simulink model "Kunal-Jain_14AE10019_MagLev"  (R2015a)
settings: Solver=ode23  StartTime=0.0  StopTime=10  RelTol=1e-3
libraries: simulink x4
settings Model: Creator=Kunal  LastModifiedBy=Kunal
settings SolverCC: AutoInsertRateTranBlk=on

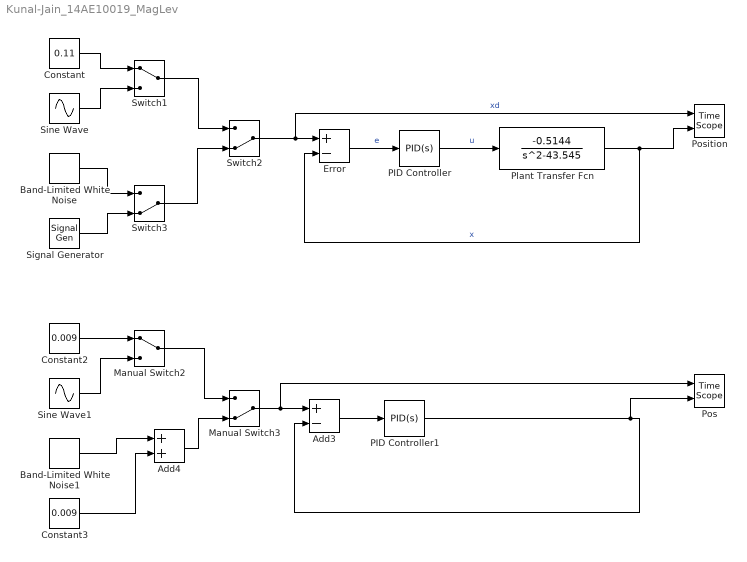
== system Kunal-Jain_14AE10019_MagLev ==
  Add3 : Sum  Inputs=+-
  Add4 : Sum
  Band-Limited White Noise : simulink/Sources/Band-Limited White Noise  Cov=[0.1]  Ts=0.1  seed=[23341]
  Band-Limited White Noise1 : simulink/Sources/Band-Limited White Noise  Cov=[0.1]  Ts=0.1  seed=[23341]
  Constant : Constant  Value=0.11
  Constant2 : Constant  Value=0.009
  Constant3 : Constant  Value=0.009
  Error : Sum  Inputs=+-
  Manual Switch2 : ManualSwitch
  Manual Switch3 : ManualSwitch  CurrentSetting=0
  PID Controller : simulink/Continuous/PID Controller  Controller=PID  TimeDomain=Continuous-time  SampleTime=-1  IntegratorMethod=Forward Euler  FilterMethod=Forward Euler  Form=Parallel  UseFilter=on  ControllerParametersSource=internal  P=-1802.63633168845  I=-5937.61734268954  D=-134.383925464391  N=383.737180014477  InitialConditionSource=internal  InitialConditionForIntegrator=0  InitialConditionForFilter=0  ExternalReset=none  LimitOutput=off  UpperSaturationLimit=inf  LowerSaturationLimit=-inf  LinearizeAsGain=on  AntiWindupMode=none  Kb=1  TrackingMode=off  Kt=1  PParamMin=[]  PParamMax=[]  IParamMin=[]  IParamMax=[]  DParamMin=[]  DParamMax=[]  NParamMin=[]  NParamMax=[]  KbParamMin=[]  KbParamMax=[]  KtParamMin=[]  KtParamMax=[]  POutMin=[]  POutMax=[]  IOutMin=[]  IOutMax=[]  DOutMin=[]  DOutMax=[]  NOutMin=[]  NOutMax=[]  KbOutMin=[]  KbOutMax=[]  KtOutMin=[]  KtOutMax=[]  IntegratorOutMin=[]  IntegratorOutMax=[]  FilterOutMin=[]  FilterOutMax=[]  SumOutMin=[]  SumOutMax=[]  SumI1OutMin=[]  SumI1OutMax=[]  SumI2OutMin=[]  SumI2OutMax=[]  SumI3OutMin=[]  SumI3OutMax=[]  SumDOutMin=[]  SumDOutMax=[]  SaturationOutMin=[]  SaturationOutMax=[]  IntegratorContinuousStateAttributes=''  IntegratorStateMustResolveToSignalObject=off  IntegratorRTWStateStorageClass=Auto  FilterContinuousStateAttributes=''  FilterStateMustResolveToSignalObject=off  FilterRTWStateStorageClass=Auto  DifferentiatorICPrevScaledInput=0  DifferentiatorOutMin=[]  DifferentiatorOutMax=[]
  PID Controller1 : simulink/Continuous/PID Controller  Controller=PID  TimeDomain=Continuous-time  SampleTime=-1  IntegratorMethod=Forward Euler  FilterMethod=Forward Euler  Form=Parallel  UseFilter=on  ControllerParametersSource=internal  P=-1802.63633168845  I=-5937.61734268954  D=-134.383925464391  N=383.737180014477  InitialConditionSource=internal  InitialConditionForIntegrator=0  InitialConditionForFilter=0  ExternalReset=none  LimitOutput=off  UpperSaturationLimit=inf  LowerSaturationLimit=-inf  LinearizeAsGain=on  AntiWindupMode=none  Kb=1  TrackingMode=off  Kt=1  PParamMin=[]  PParamMax=[]  IParamMin=[]  IParamMax=[]  DParamMin=[]  DParamMax=[]  NParamMin=[]  NParamMax=[]  KbParamMin=[]  KbParamMax=[]  KtParamMin=[]  KtParamMax=[]  POutMin=[]  POutMax=[]  IOutMin=[]  IOutMax=[]  DOutMin=[]  DOutMax=[]  NOutMin=[]  NOutMax=[]  KbOutMin=[]  KbOutMax=[]  KtOutMin=[]  KtOutMax=[]  IntegratorOutMin=[]  IntegratorOutMax=[]  FilterOutMin=[]  FilterOutMax=[]  SumOutMin=[]  SumOutMax=[]  SumI1OutMin=[]  SumI1OutMax=[]  SumI2OutMin=[]  SumI2OutMax=[]  SumI3OutMin=[]  SumI3OutMax=[]  SumDOutMin=[]  SumDOutMax=[]  SaturationOutMin=[]  SaturationOutMax=[]  IntegratorContinuousStateAttributes=''  IntegratorStateMustResolveToSignalObject=off  IntegratorRTWStateStorageClass=Auto  FilterContinuousStateAttributes=''  FilterStateMustResolveToSignalObject=off  FilterRTWStateStorageClass=Auto  DifferentiatorICPrevScaledInput=0  DifferentiatorOutMin=[]  DifferentiatorOutMax=[]
  Plant Transfer Fcn : TransferFcn  Numerator=[-0.5144]  Denominator=[1 0 -43.545]
  Pos : TimeScope  NumInputPorts=2
  Position : TimeScope  NumInputPorts=2
  Signal Generator : SignalGenerator  WaveForm=sawtooth  Amplitude=0.1  Frequency=10  Units=rad/sec
  Sine Wave : Sin  Amplitude=0.1  Frequency=10  SampleTime=0
  Sine Wave1 : Sin  SampleTime=0
  Switch1 : ManualSwitch
  Switch2 : ManualSwitch  CurrentSetting=0
  Switch3 : ManualSwitch  CurrentSetting=0
  wires:
  Error/1 -> PID Controller/1  "e"
  PID Controller/1 -> Plant Transfer Fcn/1  "u"
  Plant Transfer Fcn/1 -> Position/2, Error/2  "x"
  Constant/1 -> Switch1/1
  Switch2/1 -> Position/1, Error/1  "xd"
  Switch1/1 -> Switch2/1
  Sine Wave/1 -> Switch1/2
  Band-Limited White Noise/1 -> Switch3/1
  Add3/1 -> PID Controller1/1
  PID Controller1/1 -> Add3/2, Pos/2
  Constant2/1 -> Manual Switch2/1
  Manual Switch3/1 -> Add3/1, Pos/1
  Manual Switch2/1 -> Manual Switch3/1
  Sine Wave1/1 -> Manual Switch2/2
  Add4/1 -> Manual Switch3/2
  Band-Limited White Noise1/1 -> Add4/1
  Constant3/1 -> Add4/2
  Switch3/1 -> Switch2/2
  Signal Generator/1 -> Switch3/2
